simulink model "gm_sampleModel2019_sub"  (R2023a)
settings: Solver=VariableStepAuto  StartTime=0.0  StopTime=10.0  RelTol=1e-3
libraries: simulink x2, hdlsllib x1
settings Model: Creator=user1  LastModifiedBy=user1
settings OptimizationCC: BlockReduction=off  ConditionallyExecuteInputs=off
settings DebuggingCC: InheritedTsInSrcMsg=none

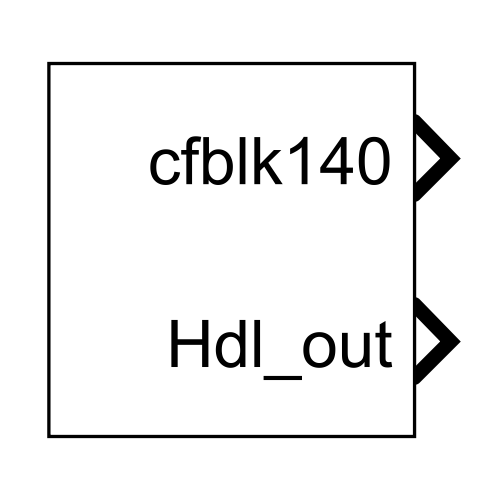
[thumbnail: Simulink's stored preview of the top-level diagram]
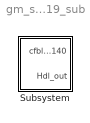
== system gm_sampleModel2019_sub ==
  Subsystem : Subsystem

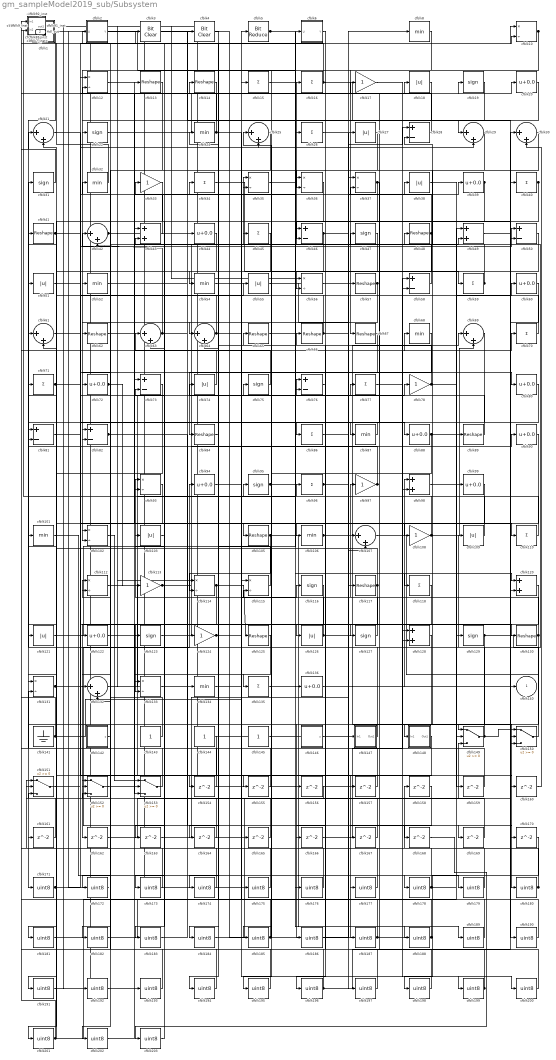
== system gm_sampleModel2019_sub/Subsystem ==
  cfblk1 : Subsystem  mask(Detect Fall Negative){vinit=double(0), InputProcessing=Elements as channels (sample based), OutDataTypeStr=uint8}
      mask prompts: vinit "Simulink:masks:InitialCondition_MP"; InputProcessing "Simulink:masks:InputProcessing_MP"; OutDataTypeStr "Simulink:masks:OutputDataType_MP"
      mask help: Simulink:masks:DetectFallNegative_MD
      mask init:
      | InputProcessing = 'Elements as channels (sample based)';
      | OutDataTypeStr = 'uint8';
      | vinit = double(0);
      mask TypeOptions InputProcessing: Simulink:masks:ColumnsAsChannelsFrameBased | Simulink:masks:ElementsAsChannelsSampleBased
      mask TypeOptions OutDataTypeStr: Simulink:masks:uint8 | Simulink:masks:boolean
      mask Display: fprintf('U < 0\n&  NOT\nU/z < 0')
  cfblk{10,12,35..37,56,93,102,112,114..115,131,133} (13 alike) : Product  Inputs=*/  OutDataTypeStr=uint8  RndMeth=Zero  SaturateOnIntegerOverflow=on
  cfblk100_inst : Subsystem
  cfblk{8,24,32,52,54,68,87,101,106,134} (10 alike) : MinMax  OutDataTypeStr=uint8
  cfblk{18,27,38,51,55,74,103,109,121,126} (10 alike) : Abs  OutDataTypeStr=uint8  SaturateOnIntegerOverflow=off
  cfblk104_inst : Subsystem
  cfblk{13..14,41,48,57,62,65..67,84,89,105,117,125,130} (15 alike) : Reshape
  cfblk{21,25,29..30,42,61,63..64,69,107,132} (11 alike) : Sum  Inputs=|++  OutDataTypeStr=uint8
  cfblk{17,33,78,97,108,113,124} (7 alike) : Gain  OutDataTypeStr=uint8
  cfblk{15..16,26,34,40,45,59,70..71,77,86,96,110,118,135} (15 alike) : Sum  Inputs=+  OutDataTypeStr=uint8
  cfblk111_inst : Subsystem
  cfblk{19,22,31,47,75,95,116,123,127,129} (10 alike) : Signum
  cfblk119_inst : Subsystem
  cfblk11_inst : Subsystem
  cfblk{43,49,98,120,128} (5 alike) : Sum  OutDataTypeStr=uint8
  cfblk{20,39,44,60,72,80,88,90,94,99,122,136} (12 alike) : Bias  Bias=0.0  SaturateOnIntegerOverflow=off
  cfblk141 : Ground
  cfblk142 : Subsystem  mask(Counter Limited){uplimit=double(7), tsamp=double(-1)}
      mask prompts: uplimit "Simulink:masks:UpperLimit_MP"; tsamp "Simulink:masks:SampleTime_MP"
      mask help: Simulink:masks:CounterLimited_MD
      mask init:
      | nbits = double(8);
      | tsamp = double(-1);
      | uplimit = double(7);
  cfblk143 : Constant  OutDataTypeStr=uint8  SampleTime=-1
  cfblk144 : Constant  OutDataTypeStr=uint8  SampleTime=-1
  cfblk145 : Constant  OutDataTypeStr=uint8  SampleTime=-1
  cfblk146 : Subsystem  mask(Counter Free-Running){NumBits=double(16), tsamp=double(-1)}
      mask prompts: NumBits "Simulink:masks:NumberOfBits_MP"; tsamp "Simulink:masks:SampleTime_MP"
      mask help: Simulink:masks:CounterFreeRunning_MD
  cfblk147 : Subsystem
  cfblk148 : Subsystem
  cfblk{149..153} (5 alike) : Switch  OutDataTypeStr=uint8  SaturateOnIntegerOverflow=off  InputSameDT=off
  cfblk{154..170} (17 alike) : Delay  SampleTime=1
  cfblk{171..203} (33 alike) : DataTypeConversion  OutDataTypeStr=uint8  SaturateOnIntegerOverflow=off  RndMeth=Floor
  cfblk2 : Subsystem  mask(Detect Rise Positive){vinit=double(0), InputProcessing=Elements as channels (sample based), OutDataTypeStr=uint8}
      mask prompts: vinit "Simulink:masks:InitialCondition_MP"; InputProcessing "Simulink:masks:InputProcessing_MP"; OutDataTypeStr "Simulink:masks:OutputDataType_MP"
      mask help: Simulink:masks:DetectRisePositive_MD
      mask init:
      | InputProcessing = 'Elements as channels (sample based)';
      | OutDataTypeStr = 'uint8';
      | vinit = double(0);
      mask TypeOptions InputProcessing: Simulink:masks:ColumnsAsChannelsFrameBased | Simulink:masks:ElementsAsChannelsSampleBased
      mask TypeOptions OutDataTypeStr: Simulink:masks:uint8 | Simulink:masks:boolean
      mask Display: fprintf('U > 0\n&  NOT\nU/z > 0')
  cfblk23_inst : Subsystem
  cfblk{28,46,50,58,73,76,81..82} (8 alike) : Sum  Inputs=+-  OutDataTypeStr=uint8
  cfblk3 : simulink/Logic and Bit Operations/Bit Clear  iBit=0
      settings: LibrarySourceBlock=|
      | hdlsllib/Logic and Bit
      | Operations/Bit Clear
  cfblk4 : simulink/Logic and Bit Operations/Bit Clear  iBit=0
      settings: LibrarySourceBlock=|
      | hdlsllib/Logic and Bit
      | Operations/Bit Clear
  cfblk5 : hdlsllib/Logic and Bit Operations/Bit Reduce  mode=AND
  cfblk53_inst : Subsystem
  cfblk6 : Subsystem  mask(Detect Fall Negative){vinit=double(0), InputProcessing=Elements as channels (sample based), OutDataTypeStr=uint8}
      mask prompts: vinit "Simulink:masks:InitialCondition_MP"; InputProcessing "Simulink:masks:InputProcessing_MP"; OutDataTypeStr "Simulink:masks:OutputDataType_MP"
      mask help: Simulink:masks:DetectFallNegative_MD
      mask init:
      | InputProcessing = 'Elements as channels (sample based)';
      | OutDataTypeStr = 'uint8';
      | vinit = double(0);
      mask TypeOptions InputProcessing: Simulink:masks:ColumnsAsChannelsFrameBased | Simulink:masks:ElementsAsChannelsSampleBased
      mask TypeOptions OutDataTypeStr: Simulink:masks:uint8 | Simulink:masks:boolean
      mask Display: fprintf('U < 0\n&  NOT\nU/z < 0')
  cfblk7_inst : Subsystem
  cfblk85_inst : Subsystem
  cfblk91_inst : Subsystem
  cfblk92_inst : Subsystem
  cfblk9_inst : Subsystem
  cfblk140 : Outport  OutDataTypeStr=uint8  SampleTime=1  VectorParamsAs1DForOutWhenUnconnected=off
  Hdl_out : Outport  Port=2  OutDataTypeStr=uint8  SampleTime=1
  wires:
  cfblk1/1(Y) -> cfblk171/1
  cfblk10/1 -> cfblk67/1, cfblk102/2
  cfblk100_inst/1(out1) -> cfblk13/1, cfblk134/1
  cfblk101/1 -> cfblk178/1
  cfblk102/1 -> cfblk153/1
  cfblk103/1 -> cfblk173/1
  cfblk104_inst/1(out1) -> cfblk44/1
  cfblk105/1 -> cfblk194/1, cfblk179/1
  cfblk106/1 -> cfblk69/1, cfblk140/1
  cfblk107/1 -> cfblk180/1
  cfblk108/1 -> cfblk69/2, cfblk53_inst/2(in2)
  cfblk109/1 -> cfblk31/1
  cfblk11_inst/1(out1) -> cfblk57/1
  cfblk110/1 -> cfblk96/1
  cfblk111_inst/1(out1) -> cfblk11_inst/2(in2), cfblk147/1(In1)
  cfblk112/1 -> cfblk187/1
  cfblk113/1 -> cfblk47/1, cfblk16/1
  cfblk114/1 -> cfblk125/1, cfblk162/1
  cfblk115/1 -> cfblk14/1
  cfblk116/1 -> cfblk135/1
  cfblk117/1 -> cfblk61/2, cfblk133/2
  cfblk118/1 -> cfblk155/1
  cfblk119_inst/1(out1) -> cfblk193/1
  cfblk12/1 -> cfblk86/1
  cfblk120/1 -> cfblk153/2
  cfblk121/1 -> cfblk26/1
  cfblk122/1 -> cfblk75/1
  cfblk123/1 -> cfblk90/1
  cfblk124/1 -> cfblk174/1, cfblk169/1
  cfblk125/1 -> cfblk153/3
  cfblk126/1 -> cfblk150/2, cfblk93/1
  cfblk127/1 -> cfblk97/1
  cfblk128/1 -> cfblk161/1
  cfblk129/1 -> cfblk48/1, cfblk186/1
  cfblk13/1 -> cfblk122/1
  cfblk130/1 -> cfblk63/2, cfblk149/1
  cfblk131/1 -> cfblk94/1, cfblk170/1
  cfblk132/1 -> cfblk6/1(U)
  cfblk133/1 -> cfblk43/2
  cfblk134/1 -> cfblk116/1
  cfblk135/1 -> cfblk188/1
  cfblk136/1 -> cfblk98/1
  cfblk14/1 -> cfblk82/2
  cfblk141/1 -> cfblk92_inst/2(in2), cfblk53_inst/1(in1), cfblk21/2, cfblk15/1
  cfblk142/1(y) -> cfblk172/1
  cfblk143/1 -> cfblk104_inst/1(in1)
  cfblk144/1 -> cfblk152/2
  cfblk145/1 -> cfblk25/1
  cfblk146/1(y) -> cfblk27/1
  cfblk147/1(Out1) -> cfblk51/1
  cfblk148/1(Out1) -> cfblk181/1
  cfblk149/1 -> cfblk66/1, cfblk150/1
  cfblk15/1 -> cfblk110/1
  cfblk150/1 -> cfblk109/1
  cfblk151/1 -> cfblk78/1
  cfblk152/1 -> cfblk68/1
  cfblk153/1 -> cfblk7_inst/2(in2)
  cfblk154/1 -> cfblk131/2
  cfblk155/1 -> cfblk133/1
  cfblk156/1 -> cfblk151/3
  cfblk157/1 -> cfblk81/2
  cfblk158/1 -> cfblk177/1
  cfblk159/1 -> cfblk35/1
  cfblk16/1 -> cfblk92_inst/1(in1), cfblk150/3, cfblk36/2
  cfblk160/1 -> cfblk30/2
  cfblk161/1 -> cfblk151/2
  cfblk162/1 -> cfblk149/3
  cfblk163/1 -> cfblk37/1
  cfblk164/1 -> cfblk42/1
  cfblk165/1 -> cfblk63/1
  cfblk166/1 -> cfblk58/1
  cfblk167/1 -> cfblk43/1
  cfblk168/1 -> cfblk203/1
  cfblk169/1 -> cfblk64/2
  cfblk17/1 -> cfblk128/1
  cfblk170/1 -> cfblk198/1
  cfblk171/1 -> cfblk55/1, cfblk50/1
  cfblk172/1 -> cfblk1/1(U)
  cfblk173/1 -> cfblk32/1
  cfblk174/1 -> cfblk103/1
  cfblk175/1 -> cfblk151/1
  cfblk176/1 -> cfblk85_inst/1(in1)
  cfblk177/1 -> cfblk85_inst/2(in2)
  cfblk178/1 -> cfblk89/1, cfblk115/2
  cfblk179/1 -> cfblk101/1
  cfblk18/1 -> cfblk98/2
  cfblk180/1 -> cfblk9_inst/2(in2), cfblk33/1, cfblk158/1
  cfblk181/1 -> cfblk107/1
  cfblk182/1 -> cfblk107/2
  cfblk183/1 -> cfblk4/1
  cfblk184/1 -> cfblk40/1
  cfblk185/1 -> cfblk65/1, cfblk11_inst/1(in1)
  cfblk186/1 -> cfblk8/1
  cfblk187/1 -> cfblk124/1, cfblk115/1
  cfblk188/1 -> cfblk112/1, Hdl_out/1
  cfblk189/1 -> cfblk112/2
  cfblk19/1 -> cfblk164/1
  cfblk190/1 -> cfblk95/1
  cfblk191/1 -> cfblk49/1
  cfblk192/1 -> cfblk49/2
  cfblk193/1 -> cfblk111_inst/1(in1)
  cfblk194/1 -> cfblk119_inst/1(in1)
  cfblk195/1 -> cfblk119_inst/2(in2)
  cfblk196/1 -> cfblk30/1, cfblk100_inst/1(in1)
  cfblk197/1 -> cfblk76/1
  cfblk198/1 -> cfblk76/2
  cfblk199/1 -> cfblk152/3, cfblk37/2
  cfblk2/1(Y) -> cfblk176/1
  cfblk20/1 -> cfblk22/1
  cfblk200/1 -> cfblk77/1
  cfblk201/1 -> cfblk41/1, cfblk117/1, cfblk111_inst/2(in2)
  cfblk202/1 -> cfblk73/1
  cfblk203/1 -> cfblk73/2
  cfblk21/1 -> cfblk160/1
  cfblk22/1 -> cfblk19/1
  cfblk23_inst/1(out1) -> cfblk157/1
  cfblk24/1 -> cfblk91_inst/2(in2), cfblk7_inst/1(in1), cfblk128/2
  cfblk25/1 -> cfblk64/1
  cfblk26/1 -> cfblk59/1
  cfblk27/1 -> cfblk62/1
  cfblk28/1 -> cfblk12/2
  cfblk29/1 -> cfblk148/1(In1)
  cfblk3/1 -> cfblk29/1
  cfblk30/1 -> cfblk72/1
  cfblk31/1 -> cfblk104_inst/2(in2)
  cfblk32/1 -> cfblk9_inst/1(in1)
  cfblk33/1 -> cfblk191/1
  cfblk34/1 -> cfblk136/1
  cfblk35/1 -> cfblk130/1
  cfblk36/1 -> cfblk163/1
  cfblk37/1 -> cfblk132/2, cfblk87/1
  cfblk38/1 -> cfblk159/1
  cfblk39/1 -> cfblk46/2, cfblk52/1
  cfblk4/1 -> cfblk184/1
  cfblk40/1 -> cfblk152/1, cfblk149/2
  cfblk41/1 -> cfblk80/1, cfblk127/1
  cfblk42/1 -> cfblk20/1, cfblk108/1
  cfblk43/1 -> cfblk12/1
  cfblk44/1 -> cfblk93/2
  cfblk45/1 -> cfblk123/1
  cfblk46/1 -> cfblk120/1, cfblk114/2
  cfblk47/1 -> cfblk121/1
  cfblk48/1 -> cfblk3/1, cfblk54/1
  cfblk49/1 -> cfblk190/1
  cfblk5/1 -> cfblk58/2, cfblk50/2
  cfblk50/1 -> cfblk126/1
  cfblk51/1 -> cfblk10/2
  cfblk52/1 -> cfblk29/2
  cfblk53_inst/1(out1) -> cfblk165/1
  cfblk54/1 -> cfblk5/1
  cfblk55/1 -> cfblk197/1
  cfblk56/1 -> cfblk10/1
  cfblk57/1 -> cfblk82/1, cfblk182/1
  cfblk58/1 -> cfblk35/2
  cfblk59/1 -> cfblk91_inst/1(in1), cfblk28/2
  cfblk6/1(Y) -> cfblk56/2
  cfblk60/1 -> cfblk120/2
  cfblk61/1 -> cfblk106/1
  cfblk62/1 -> cfblk34/1
  cfblk63/1 -> cfblk42/2, cfblk36/1
  cfblk64/1 -> cfblk46/1, cfblk2/1(U)
  cfblk65/1 -> cfblk189/1
  cfblk66/1 -> cfblk38/1, cfblk21/1, cfblk24/1
  cfblk67/1 -> cfblk166/1
  cfblk68/1 -> cfblk84/1
  cfblk69/1 -> cfblk132/1
  cfblk7_inst/1(out1) -> cfblk192/1
  cfblk70/1 -> cfblk45/1
  cfblk71/1 -> cfblk88/1, cfblk18/1
  cfblk72/1 -> cfblk202/1, cfblk113/1
  cfblk73/1 -> cfblk201/1
  cfblk74/1 -> cfblk23_inst/2(in2)
  cfblk75/1 -> cfblk61/1
  cfblk76/1 -> cfblk196/1
  cfblk77/1 -> cfblk199/1
  cfblk78/1 -> cfblk129/1, cfblk100_inst/2(in2)
  cfblk8/1 -> cfblk185/1
  cfblk80/1 -> cfblk105/1
  cfblk81/1 -> cfblk25/2
  cfblk82/1 -> cfblk168/1, cfblk167/1
  cfblk84/1 -> cfblk154/1
  cfblk85_inst/1(out1) -> cfblk175/1
  cfblk86/1 -> cfblk70/1
  cfblk87/1 -> cfblk81/1
  cfblk88/1 -> cfblk60/1, cfblk195/1
  cfblk89/1 -> cfblk74/1
  cfblk9_inst/1(out1) -> cfblk23_inst/1(in1)
  cfblk90/1 -> cfblk131/1
  cfblk91_inst/1(out1) -> cfblk114/1
  cfblk92_inst/1(out1) -> cfblk56/1
  cfblk93/1 -> cfblk102/1
  cfblk94/1 -> cfblk200/1
  cfblk95/1 -> cfblk156/1, cfblk118/1
  cfblk96/1 -> cfblk39/1, cfblk28/1
  cfblk97/1 -> cfblk17/1, cfblk71/1
  cfblk98/1 -> cfblk99/1
  cfblk99/1 -> cfblk183/1

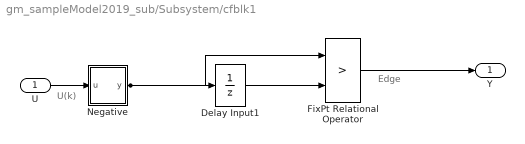
== system gm_sampleModel2019_sub/Subsystem/cfblk1 ==
  note: U(k)
  note: Edge
  U : Inport  OutDataTypeStr=uint8  SampleTime=1
  Delay Input1 : UnitDelay  Description=Store in Global RAM  DisableCoverage=on  InitialCondition=vinit  SampleTime=-1  HasFrameUpgradeWarning=on
  FixPt Relational Operator : RelationalOperator  Operator=>  OutDataTypeStr=fixdt(0, 8)  ZeroCross=off  InputSameDT=off
  Negative : Subsystem  mask(Compare To Zero){relop=<, OutDataTypeStr=boolean, ZeroCross=off}
      mask prompts: relop "Simulink:masks:Operator_MP"; OutDataTypeStr "Simulink:masks:OutputDataType_MP"; ZeroCross "Simulink:masks:EnableZerocrossingDetection_MP"
      mask help: Simulink:masks:CompareToZero_MD
      mask init:
      | OutDataTypeStr = 'boolean';
      | ZeroCross = 'off';
      | blkName = 'sampleModel2019_sub/Subsystem/cfblk1/Negative';
      | relop = '<';
      | setValue = 'boolean';
      mask TypeOptions relop: == | ~= | < | <= | >= | >
      mask TypeOptions OutDataTypeStr: Simulink:masks:uint8 | Simulink:masks:boolean
      mask Callback ZeroCross: sl('zeroCrossEnable', gcbh);
      mask Display: disp([relop,' 0'])
  Y : Outport  SampleTime=1
  wires:
  U/1 -> Negative/1(u)
  Delay Input1/1 -> FixPt Relational Operator/2
  FixPt Relational Operator/1 -> Y/1
  Negative/1(y) -> FixPt Relational Operator/1, Delay Input1/1

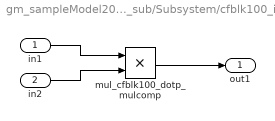
== system gm_sampleModel2019_sub/Subsystem/cfblk100_inst ==
  in1 : Inport  OutDataTypeStr=uint8  SampleTime=1
  in2 : Inport  Port=2  OutDataTypeStr=uint8  SampleTime=1
  mul_cfblk100_dotp_mulcomp : Product  Inputs=**  OutDataTypeStr=uint8  SampleTime=1
  out1 : Outport  OutDataTypeStr=uint8  SampleTime=1
  wires:
  in1/1 -> mul_cfblk100_dotp_mulcomp/1
  in2/1 -> mul_cfblk100_dotp_mulcomp/2
  mul_cfblk100_dotp_mulcomp/1 -> out1/1

== system gm_sampleModel2019_sub/Subsystem/cfblk104_inst ==
  in1 : Inport  OutDataTypeStr=uint8  SampleTime=1
  in2 : Inport  Port=2  OutDataTypeStr=uint8  SampleTime=1
  mul_cfblk104_dotp_mulcomp : Product  Inputs=**  OutDataTypeStr=uint8  SampleTime=1
  out1 : Outport  OutDataTypeStr=uint8  SampleTime=1
  wires:
  in1/1 -> mul_cfblk104_dotp_mulcomp/1
  in2/1 -> mul_cfblk104_dotp_mulcomp/2
  mul_cfblk104_dotp_mulcomp/1 -> out1/1

== system gm_sampleModel2019_sub/Subsystem/cfblk111_inst ==
  in1 : Inport  OutDataTypeStr=uint8  SampleTime=1
  in2 : Inport  Port=2  OutDataTypeStr=uint8  SampleTime=1
  mul_cfblk111_dotp_mulcomp : Product  Inputs=**  OutDataTypeStr=uint8  SampleTime=1
  out1 : Outport  OutDataTypeStr=uint8  SampleTime=1
  wires:
  in1/1 -> mul_cfblk111_dotp_mulcomp/1
  in2/1 -> mul_cfblk111_dotp_mulcomp/2
  mul_cfblk111_dotp_mulcomp/1 -> out1/1

== system gm_sampleModel2019_sub/Subsystem/cfblk119_inst ==
  in1 : Inport  OutDataTypeStr=uint8  SampleTime=1
  in2 : Inport  Port=2  OutDataTypeStr=uint8  SampleTime=1
  mul_cfblk119_dotp_mulcomp : Product  Inputs=**  OutDataTypeStr=uint8  SampleTime=1
  out1 : Outport  OutDataTypeStr=uint8  SampleTime=1
  wires:
  in1/1 -> mul_cfblk119_dotp_mulcomp/1
  in2/1 -> mul_cfblk119_dotp_mulcomp/2
  mul_cfblk119_dotp_mulcomp/1 -> out1/1

== system gm_sampleModel2019_sub/Subsystem/cfblk11_inst ==
  in1 : Inport  OutDataTypeStr=uint8  SampleTime=1
  in2 : Inport  Port=2  OutDataTypeStr=uint8  SampleTime=1
  mul_cfblk11_dotp_mulcomp : Product  Inputs=**  OutDataTypeStr=uint8  SampleTime=1
  out1 : Outport  OutDataTypeStr=uint8  SampleTime=1
  wires:
  in1/1 -> mul_cfblk11_dotp_mulcomp/1
  in2/1 -> mul_cfblk11_dotp_mulcomp/2
  mul_cfblk11_dotp_mulcomp/1 -> out1/1

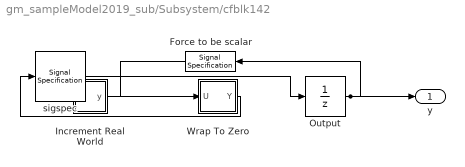
== system gm_sampleModel2019_sub/Subsystem/cfblk142 ==
  Force to be scalar : SignalSpecification  DisableCoverage=on  Dimensions=1
  Increment Real World : Subsystem  mask(Real World Value Increment){}
      mask help: Simulink:masks:RealWorldValueIncrement_MD
      mask Display: disp('V++')
  Output : UnitDelay  InitialCondition=0.0  SampleTime=tsamp  HasFrameUpgradeWarning=on
  Wrap To Zero : Subsystem  mask(Wrap To Zero){Threshold=double(7)}
      mask prompts: Threshold "Simulink:masks:Threshold_MP"
      mask help: Simulink:masks:WrapToZero_MD
  sigspec : SignalSpecification  OutDataTypeStr=uint8  Dimensions=1
  y : Outport  SampleTime=1
  wires:
  Force to be scalar/1 -> Increment Real World/1(u)
  Increment Real World/1(y) -> Wrap To Zero/1(U)
  Output/1 -> Force to be scalar/1, y/1
  Wrap To Zero/1(Y) -> sigspec/1
  sigspec/1 -> Output/1

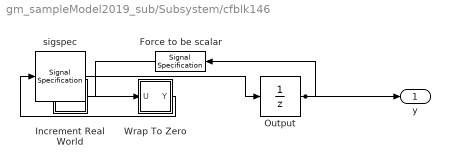
== system gm_sampleModel2019_sub/Subsystem/cfblk146 ==
  Force to be scalar : SignalSpecification  DisableCoverage=on  Dimensions=1
  Increment Real World : Subsystem  mask(Real World Value Increment){}
      mask help: Simulink:masks:RealWorldValueIncrement_MD
      mask Display: disp('V++')
  Output : UnitDelay  InitialCondition=0.0  SampleTime=tsamp  HasFrameUpgradeWarning=on
  Wrap To Zero : Subsystem  mask(Wrap To Zero){Threshold=double(65535)}
      mask prompts: Threshold "Simulink:masks:Threshold_MP"
      mask help: Simulink:masks:WrapToZero_MD
  sigspec : SignalSpecification  OutDataTypeStr=uint16  Dimensions=1
  y : Outport  SampleTime=1
  wires:
  Force to be scalar/1 -> Increment Real World/1(u)
  Increment Real World/1(y) -> Wrap To Zero/1(U)
  Output/1 -> Force to be scalar/1, y/1
  Wrap To Zero/1(Y) -> sigspec/1
  sigspec/1 -> Output/1

== system gm_sampleModel2019_sub/Subsystem/cfblk147 ==
  In1 : Inport  OutDataTypeStr=uint8  PortDimensions=1  SampleTime=1
  Out1 : Outport  SampleTime=1
  wires:
  In1/1 -> Out1/1

== system gm_sampleModel2019_sub/Subsystem/cfblk148 ==
  In1 : Inport  OutDataTypeStr=uint8  PortDimensions=1  SampleTime=1
  Out1 : Outport  SampleTime=1
  wires:
  In1/1 -> Out1/1

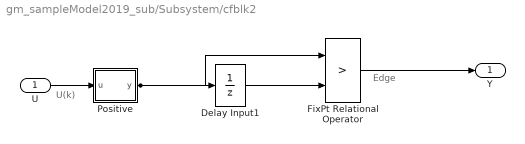
== system gm_sampleModel2019_sub/Subsystem/cfblk2 ==
  note: U(k)
  note: Edge
  U : Inport  OutDataTypeStr=uint8  SampleTime=1
  Delay Input1 : UnitDelay  Description=Store in Global RAM  DisableCoverage=on  InitialCondition=vinit  SampleTime=-1  HasFrameUpgradeWarning=on
  FixPt Relational Operator : RelationalOperator  Operator=>  OutDataTypeStr=fixdt(0, 8)  ZeroCross=off  InputSameDT=off
  Positive : Subsystem  mask(Compare To Zero){relop=>, OutDataTypeStr=boolean, ZeroCross=off}
      mask prompts: relop "Simulink:masks:Operator_MP"; OutDataTypeStr "Simulink:masks:OutputDataType_MP"; ZeroCross "Simulink:masks:EnableZerocrossingDetection_MP"
      mask help: Simulink:masks:CompareToZero_MD
      mask init:
      | OutDataTypeStr = 'boolean';
      | ZeroCross = 'off';
      | blkName = 'sampleModel2019_sub/Subsystem/cfblk2/Positive';
      | relop = '>';
      | setValue = 'boolean';
      mask TypeOptions relop: == | ~= | < | <= | >= | >
      mask TypeOptions OutDataTypeStr: Simulink:masks:uint8 | Simulink:masks:boolean
      mask Callback ZeroCross: sl('zeroCrossEnable', gcbh);
      mask Display: disp([relop,' 0'])
  Y : Outport  SampleTime=1
  wires:
  U/1 -> Positive/1(u)
  Delay Input1/1 -> FixPt Relational Operator/2
  FixPt Relational Operator/1 -> Y/1
  Positive/1(y) -> FixPt Relational Operator/1, Delay Input1/1

== system gm_sampleModel2019_sub/Subsystem/cfblk23_inst ==
  in1 : Inport  OutDataTypeStr=uint8  SampleTime=1
  in2 : Inport  Port=2  OutDataTypeStr=uint8  SampleTime=1
  mul_cfblk23_dotp_mulcomp : Product  Inputs=**  OutDataTypeStr=uint8  SampleTime=1
  out1 : Outport  OutDataTypeStr=uint8  SampleTime=1
  wires:
  in1/1 -> mul_cfblk23_dotp_mulcomp/1
  in2/1 -> mul_cfblk23_dotp_mulcomp/2
  mul_cfblk23_dotp_mulcomp/1 -> out1/1

== system gm_sampleModel2019_sub/Subsystem/cfblk53_inst ==
  in1 : Inport  OutDataTypeStr=uint8  SampleTime=1
  in2 : Inport  Port=2  OutDataTypeStr=uint8  SampleTime=1
  mul_cfblk53_dotp_mulcomp : Product  Inputs=**  OutDataTypeStr=uint8  SampleTime=1
  out1 : Outport  OutDataTypeStr=uint8  SampleTime=1
  wires:
  in1/1 -> mul_cfblk53_dotp_mulcomp/1
  in2/1 -> mul_cfblk53_dotp_mulcomp/2
  mul_cfblk53_dotp_mulcomp/1 -> out1/1

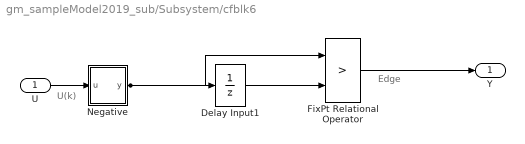
== system gm_sampleModel2019_sub/Subsystem/cfblk6 ==
  note: U(k)
  note: Edge
  U : Inport  OutDataTypeStr=uint8  SampleTime=1
  Delay Input1 : UnitDelay  Description=Store in Global RAM  DisableCoverage=on  InitialCondition=vinit  SampleTime=-1  HasFrameUpgradeWarning=on
  FixPt Relational Operator : RelationalOperator  Operator=>  OutDataTypeStr=fixdt(0, 8)  ZeroCross=off  InputSameDT=off
  Negative : Subsystem  mask(Compare To Zero){relop=<, OutDataTypeStr=boolean, ZeroCross=off}
      mask prompts: relop "Simulink:masks:Operator_MP"; OutDataTypeStr "Simulink:masks:OutputDataType_MP"; ZeroCross "Simulink:masks:EnableZerocrossingDetection_MP"
      mask help: Simulink:masks:CompareToZero_MD
      mask init:
      | OutDataTypeStr = 'boolean';
      | ZeroCross = 'off';
      | blkName = 'sampleModel2019_sub/Subsystem/cfblk6/Negative';
      | relop = '<';
      | setValue = 'boolean';
      mask TypeOptions relop: == | ~= | < | <= | >= | >
      mask TypeOptions OutDataTypeStr: Simulink:masks:uint8 | Simulink:masks:boolean
      mask Callback ZeroCross: sl('zeroCrossEnable', gcbh);
      mask Display: disp([relop,' 0'])
  Y : Outport  SampleTime=1
  wires:
  U/1 -> Negative/1(u)
  Delay Input1/1 -> FixPt Relational Operator/2
  FixPt Relational Operator/1 -> Y/1
  Negative/1(y) -> FixPt Relational Operator/1, Delay Input1/1

== system gm_sampleModel2019_sub/Subsystem/cfblk7_inst ==
  in1 : Inport  OutDataTypeStr=uint8  SampleTime=1
  in2 : Inport  Port=2  OutDataTypeStr=uint8  SampleTime=1
  mul_cfblk7_dotp_mulcomp : Product  Inputs=**  OutDataTypeStr=uint8  SampleTime=1
  out1 : Outport  OutDataTypeStr=uint8  SampleTime=1
  wires:
  in1/1 -> mul_cfblk7_dotp_mulcomp/1
  in2/1 -> mul_cfblk7_dotp_mulcomp/2
  mul_cfblk7_dotp_mulcomp/1 -> out1/1

== system gm_sampleModel2019_sub/Subsystem/cfblk85_inst ==
  in1 : Inport  OutDataTypeStr=uint8  SampleTime=1
  in2 : Inport  Port=2  OutDataTypeStr=uint8  SampleTime=1
  mul_cfblk85_dotp_mulcomp : Product  Inputs=**  OutDataTypeStr=uint8  SampleTime=1
  out1 : Outport  OutDataTypeStr=uint8  SampleTime=1
  wires:
  in1/1 -> mul_cfblk85_dotp_mulcomp/1
  in2/1 -> mul_cfblk85_dotp_mulcomp/2
  mul_cfblk85_dotp_mulcomp/1 -> out1/1

== system gm_sampleModel2019_sub/Subsystem/cfblk91_inst ==
  in1 : Inport  OutDataTypeStr=uint8  SampleTime=1
  in2 : Inport  Port=2  OutDataTypeStr=uint8  SampleTime=1
  mul_cfblk91_dotp_mulcomp : Product  Inputs=**  OutDataTypeStr=uint8  SampleTime=1
  out1 : Outport  OutDataTypeStr=uint8  SampleTime=1
  wires:
  in1/1 -> mul_cfblk91_dotp_mulcomp/1
  in2/1 -> mul_cfblk91_dotp_mulcomp/2
  mul_cfblk91_dotp_mulcomp/1 -> out1/1

== system gm_sampleModel2019_sub/Subsystem/cfblk92_inst ==
  in1 : Inport  OutDataTypeStr=uint8  SampleTime=1
  in2 : Inport  Port=2  OutDataTypeStr=uint8  SampleTime=1
  mul_cfblk92_dotp_mulcomp : Product  Inputs=**  OutDataTypeStr=uint8  SampleTime=1
  out1 : Outport  OutDataTypeStr=uint8  SampleTime=1
  wires:
  in1/1 -> mul_cfblk92_dotp_mulcomp/1
  in2/1 -> mul_cfblk92_dotp_mulcomp/2
  mul_cfblk92_dotp_mulcomp/1 -> out1/1

== system gm_sampleModel2019_sub/Subsystem/cfblk9_inst ==
  in1 : Inport  OutDataTypeStr=uint8  SampleTime=1
  in2 : Inport  Port=2  OutDataTypeStr=uint8  SampleTime=1
  mul_cfblk9_dotp_mulcomp : Product  Inputs=**  OutDataTypeStr=uint8  SampleTime=1
  out1 : Outport  OutDataTypeStr=uint8  SampleTime=1
  wires:
  in1/1 -> mul_cfblk9_dotp_mulcomp/1
  in2/1 -> mul_cfblk9_dotp_mulcomp/2
  mul_cfblk9_dotp_mulcomp/1 -> out1/1

== system gm_sampleModel2019_sub/Subsystem/cfblk1/Negative ==
  u : Inport  OutDataTypeStr=uint8  SampleTime=1
  Compare : RelationalOperator  Operator=<  OutDataTypeStr=boolean  ZeroCross=off
  Constant : Constant  DisableCoverage=on  Value=0  OutDataTypeStr=Inherit: Inherit via back propagation  SampleTime=-1  PreserveConstantTs=on
  y : Outport  SampleTime=1
  wires:
  u/1 -> Compare/1
  Compare/1 -> y/1
  Constant/1 -> Compare/2

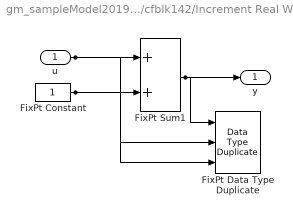
== system gm_sampleModel2019_sub/Subsystem/cfblk142/Increment Real World ==
  u : Inport  OutDataTypeStr=uint8  SampleTime=1
  FixPt Constant : Constant  DisableCoverage=on  OutDataTypeStr=Inherit: Inherit via back propagation  SampleTime=-1
  FixPt Data Type Duplicate : DataTypeDuplicate  DisableCoverage=on  NumInputPorts=3
  FixPt Sum1 : Sum  InputSameDT=on  OutDataTypeStr=Inherit: Inherit via back propagation  LockScale=on
  y : Outport  SampleTime=1
  wires:
  u/1 -> FixPt Sum1/1, FixPt Data Type Duplicate/2
  FixPt Constant/1 -> FixPt Sum1/2, FixPt Data Type Duplicate/3
  FixPt Sum1/1 -> FixPt Data Type Duplicate/1, y/1

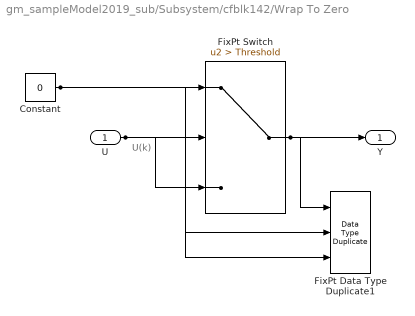
== system gm_sampleModel2019_sub/Subsystem/cfblk142/Wrap To Zero ==
  note: U(k)
  U : Inport  OutDataTypeStr=uint8  SampleTime=1
  Constant : Constant  DisableCoverage=on  Value=0  OutDataTypeStr=Inherit: Inherit via back propagation  SampleTime=-1
  FixPt Data Type Duplicate1 : DataTypeDuplicate  DisableCoverage=on  NumInputPorts=3
  FixPt Switch : Switch  Criteria=u2 > Threshold  Threshold=Threshold  OutDataTypeStr=Inherit: Inherit via back propagation  ZeroCross=off  SaturateOnIntegerOverflow=off  InputSameDT=off
  Y : Outport  SampleTime=1
  wires:
  U/1 -> FixPt Switch/3, FixPt Switch/2, FixPt Data Type Duplicate1/2
  Constant/1 -> FixPt Switch/1, FixPt Data Type Duplicate1/3
  FixPt Switch/1 -> FixPt Data Type Duplicate1/1, Y/1

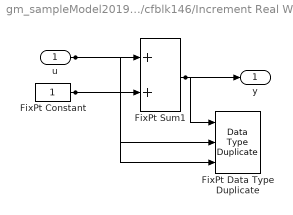
== system gm_sampleModel2019_sub/Subsystem/cfblk146/Increment Real World ==
  u : Inport  OutDataTypeStr=uint16  SampleTime=1
  FixPt Constant : Constant  DisableCoverage=on  OutDataTypeStr=Inherit: Inherit via back propagation  SampleTime=-1
  FixPt Data Type Duplicate : DataTypeDuplicate  DisableCoverage=on  NumInputPorts=3
  FixPt Sum1 : Sum  InputSameDT=on  OutDataTypeStr=Inherit: Inherit via back propagation  LockScale=on
  y : Outport  SampleTime=1
  wires:
  u/1 -> FixPt Sum1/1, FixPt Data Type Duplicate/2
  FixPt Constant/1 -> FixPt Sum1/2, FixPt Data Type Duplicate/3
  FixPt Sum1/1 -> FixPt Data Type Duplicate/1, y/1

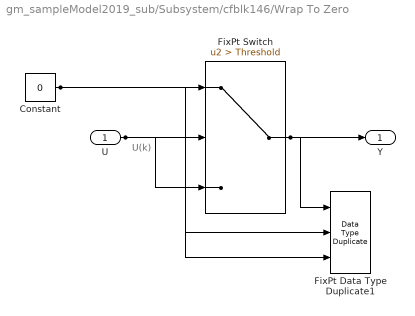
== system gm_sampleModel2019_sub/Subsystem/cfblk146/Wrap To Zero ==
  note: U(k)
  U : Inport  OutDataTypeStr=uint16  SampleTime=1
  Constant : Constant  DisableCoverage=on  Value=0  OutDataTypeStr=Inherit: Inherit via back propagation  SampleTime=-1
  FixPt Data Type Duplicate1 : DataTypeDuplicate  DisableCoverage=on  NumInputPorts=3
  FixPt Switch : Switch  Criteria=u2 > Threshold  Threshold=Threshold  OutDataTypeStr=Inherit: Inherit via back propagation  ZeroCross=off  SaturateOnIntegerOverflow=off  InputSameDT=off
  Y : Outport  SampleTime=1
  wires:
  U/1 -> FixPt Switch/3, FixPt Switch/2, FixPt Data Type Duplicate1/2
  Constant/1 -> FixPt Switch/1, FixPt Data Type Duplicate1/3
  FixPt Switch/1 -> FixPt Data Type Duplicate1/1, Y/1

== system gm_sampleModel2019_sub/Subsystem/cfblk2/Positive ==
  u : Inport  OutDataTypeStr=uint8  SampleTime=1
  Compare : RelationalOperator  Operator=>  OutDataTypeStr=boolean  ZeroCross=off
  Constant : Constant  DisableCoverage=on  Value=0  OutDataTypeStr=Inherit: Inherit via back propagation  SampleTime=-1  PreserveConstantTs=on
  y : Outport  SampleTime=1
  wires:
  u/1 -> Compare/1
  Compare/1 -> y/1
  Constant/1 -> Compare/2

== system gm_sampleModel2019_sub/Subsystem/cfblk6/Negative ==
  u : Inport  OutDataTypeStr=uint8  SampleTime=1
  Compare : RelationalOperator  Operator=<  OutDataTypeStr=boolean  ZeroCross=off
  Constant : Constant  DisableCoverage=on  Value=0  OutDataTypeStr=Inherit: Inherit via back propagation  SampleTime=-1  PreserveConstantTs=on
  y : Outport  SampleTime=1
  wires:
  u/1 -> Compare/1
  Compare/1 -> y/1
  Constant/1 -> Compare/2
